simulink model "Slide18"  (R2015b)
settings: Solver=VariableStepAuto  StartTime=0.0  StopTime=10.0  RelTol=1e-3
libraries: simulink x3
settings Model: Creator=Pouya  LastModifiedBy=Pouya

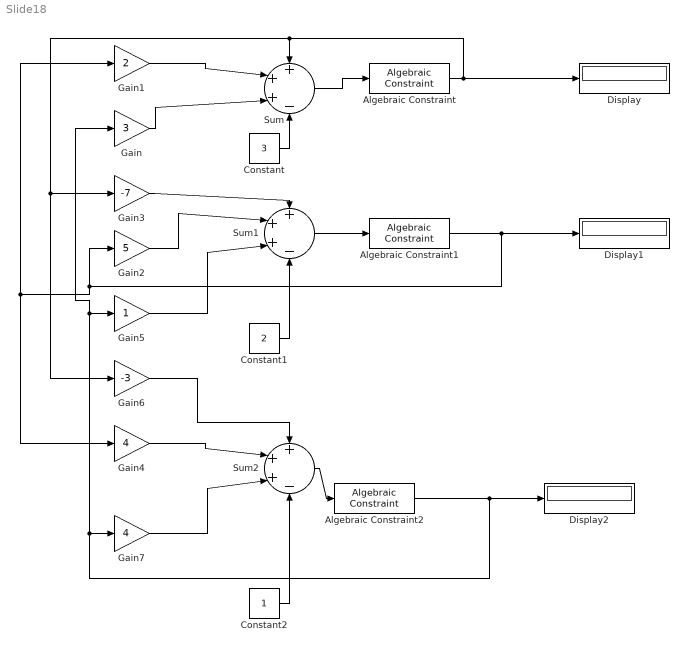
== system Slide18 ==
  Algebraic Constraint : simulink/Math Operations/Algebraic Constraint  z0=0
  Algebraic Constraint1 : simulink/Math Operations/Algebraic Constraint  z0=0
  Algebraic Constraint2 : simulink/Math Operations/Algebraic Constraint  z0=0
  Constant : Constant  Value=3
  Constant1 : Constant  Value=2
  Constant2 : Constant
  Display : Display
  Display1 : Display
  Display2 : Display
  Gain : Gain  Gain=3
  Gain1 : Gain  Gain=2
  Gain2 : Gain  Gain=5
  Gain3 : Gain  Gain=-7
  Gain4 : Gain  Gain=4
  Gain5 : Gain
  Gain6 : Gain  Gain=-3
  Gain7 : Gain  Gain=4
  Sum : Sum  Inputs=+++-
  Sum1 : Sum  Inputs=+++-
  Sum2 : Sum  Inputs=+++-
  wires:
  Algebraic Constraint/1 -> Display/1, Gain6/1, Gain3/1, Sum/1
  Algebraic Constraint1/1 -> Gain2/1, Gain4/1, Gain1/1, Display1/1
  Algebraic Constraint2/1 -> Gain/1, Gain5/1, Gain7/1, Display2/1
  Sum2/1 -> Algebraic Constraint2/1
  Sum1/1 -> Algebraic Constraint1/1
  Sum/1 -> Algebraic Constraint/1
  Gain1/1 -> Sum/2
  Gain/1 -> Sum/3
  Constant/1 -> Sum/4
  Gain3/1 -> Sum1/1
  Gain2/1 -> Sum1/2
  Constant1/1 -> Sum1/4
  Gain6/1 -> Sum2/1
  Constant2/1 -> Sum2/4
  Gain4/1 -> Sum2/2
  Gain7/1 -> Sum2/3
  Gain5/1 -> Sum1/3
